simulink model "eg7"  (R2015a)
settings: Solver=ode45  StartTime=0.0  StopTime=10.0  RelTol=1e-3
settings Model: Creator=ayush  LastModifiedBy=ayush

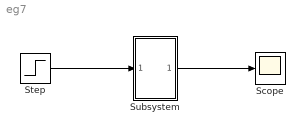
== system eg7 ==
  Scope : Scope
  Step : Step  Time=0  After=400  SampleTime=0
  Subsystem : Subsystem
  wires:
  Step/1 -> Subsystem/1(In1)
  Subsystem/1(Out1) -> Scope/1

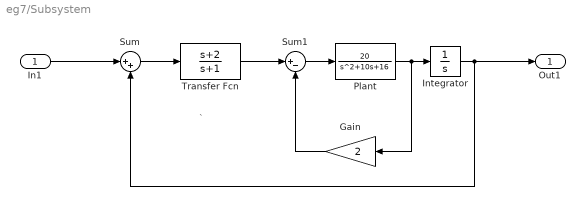
== system eg7/Subsystem ==
  note: `
  In1 : Inport
  Gain : Gain  Gain=2
  Integrator : Integrator
  Plant : TransferFcn  Numerator=[20]  Denominator=[1 10 16]
  Sum : Sum  Inputs=|++
  Sum1 : Sum  Inputs=|+-
  Transfer Fcn : TransferFcn  Numerator=[1 2]  Denominator=[1 1]
  Out1 : Outport
  wires:
  Transfer Fcn/1 -> Sum1/1
  Sum/1 -> Transfer Fcn/1
  Gain/1 -> Sum1/2
  Sum1/1 -> Plant/1
  Integrator/1 -> Out1/1, Sum/2
  In1/1 -> Sum/1
  Plant/1 -> Gain/1, Integrator/1
